simulink model "serial_interface"  (R2015a)
settings: Solver=ode3  StartTime=0.0  StopTime=inf  FixedStep=0.0001  RelTol=1e-3
undefined symbols (not defined in the file or in its folder): serial
libraries: instrumentlib x2
settings Model: SimulationMode=accelerator  Creator=rblan  LastModifiedBy=rblan

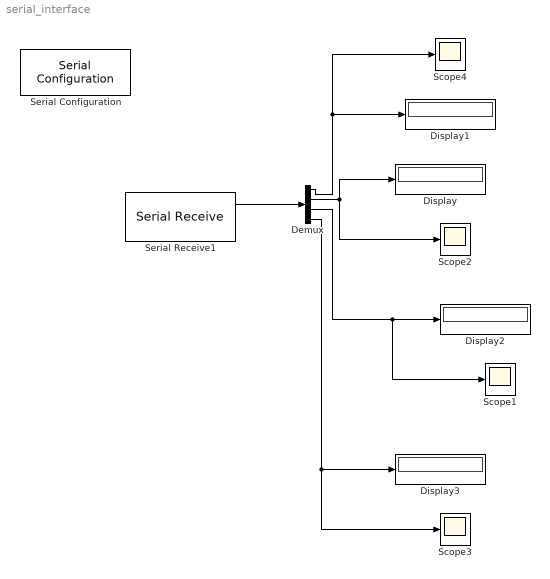
== system serial_interface ==
  Demux : Demux
  Display{,1..3} (4 alike) : Display
  Scope{1..4} (4 alike) : Scope
      Scope1 settings: YMin=-0.145  YMax=-0.09  MaxDataPoints=500000
      Scope2 settings: YMin=-20.5884  YMax=-18.6276  SaveName=ScopeData2  MaxDataPoints=5000000
      Scope3 settings: YMin=-0.3  YMax=2  MaxDataPoints=5000000
      Scope4 settings: YMin=9.69818  YMax=9.69818  SaveName=ScopeData3  MaxDataPoints=500000
  Serial Configuration : instrumentlib/Serial Configuration  Priority=-200000  ComPortMenu=<Please select a port...>  ComPort=COM3  ObjConstructor=serial('COM3');  BaudRate=9600  DataBits=8  Parity=none  StopBits=1  FlowControl=none  Timeout=10  ByteOrder=BigEndian
  Serial Receive1 : instrumentlib/Serial Receive  ComPortMenu=<Please select a port...>  ComPort=COM3  ObjConstructor=serial('COM3');  Terminator=<none>  DataSize="[4  1]"  DataType=single  EnableBlockingMode=off  ActionDataUnavailable=Output last received value  CustomValue=0  SampleTime=0.0001
  wires:
  Demux/1 -> Scope4/1, Display1/1
  Demux/2 -> Scope2/1, Display/1
  Serial Receive1/1 -> Demux/1
  Demux/3 -> Scope1/1, Display2/1
  Demux/4 -> Display3/1, Scope3/1
